simulink model "Kalman_compatible"  (R2021a)
settings: Solver=VariableStepAuto  StartTime=0.0  StopTime=10.0  RelTol=1e-3
values from neighbouring files (symbols this model uses):
  all_cov = cov(all_data)    [Analyze.m]
  ff = 1.1    [Analyze.m]
  g = 9.8    [Analyze.m]
  ground_alt = mean(z_hypsometric(ground_pressure))    [Analyze.m]
  T_s = 1/f_s    (= 0.005)    [Analyze.m]
undefined symbols (not defined in the file or in its folder): Aileron_A, Aileron_B, Discrete, Elevator_A, Elevator_B, Time
libraries: ctrlSharedLib x8
settings Model: Creator=jtc12  LastModifiedBy=Willi

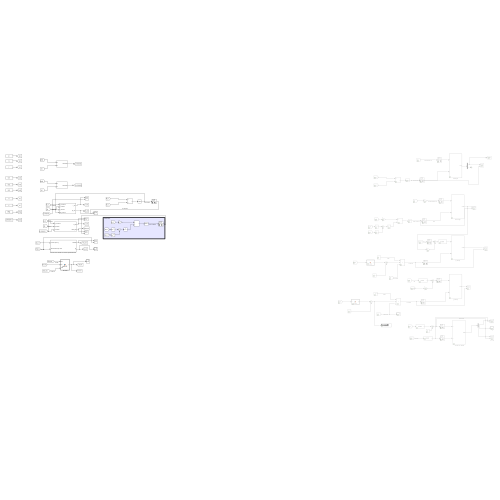
[thumbnail: Simulink's stored preview of the top-level diagram]
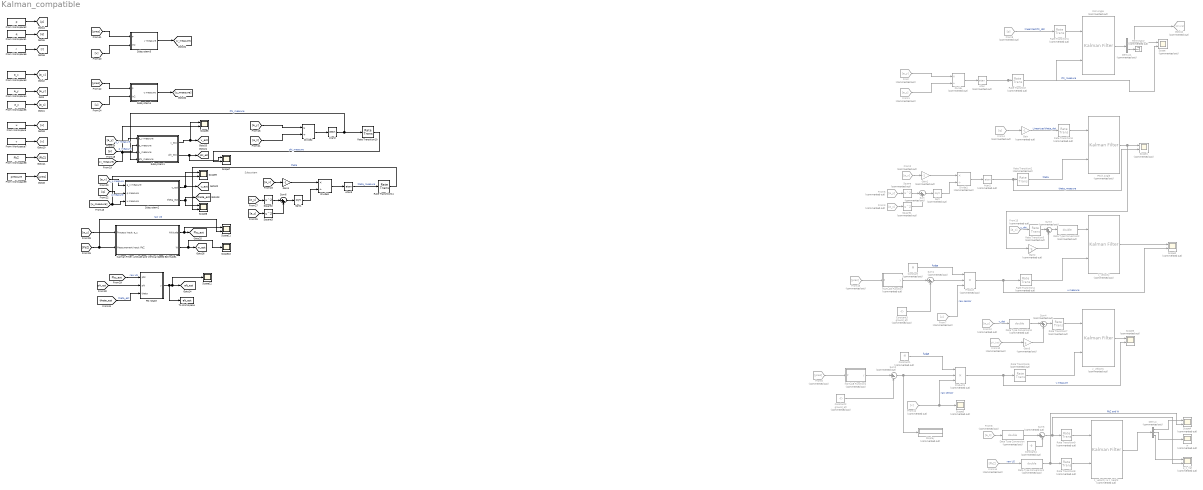
== system Kalman_compatible ==
  note: Subsystem
  Atan : Trigonometry  Commented=on  Operator=atan
  Atan1 : Trigonometry  Commented=on  Operator=atan
  Atan2 : Trigonometry  Operator=atan
  Atan3 : Trigonometry  Operator=atan
  Constant : Constant  Commented=on  Value=ff
  Constant1 : Constant  Commented=on  Value=ff
  Constant2 : Constant  Commented=on  Value=ground_alt
  Constant3 : Constant  Commented=on  Value=ground_alt
  Constant4 : Constant  Commented=on  Value=-9
  Data Type Conversion{,1..3} (4 alike) : DataTypeConversion  Commented=on  OutDataTypeStr=double
  Demux : Demux  Commented=on  Outputs=3
  Demux1 : Demux  Commented=on  Outputs=2
  Display : Display  Commented=on
  Divide : Product  Commented=on  Inputs=*/
  Divide1 : Product  Commented=on  Inputs=*/
  Divide2 : Product  Inputs=*/
  Divide3 : Product  Inputs=*/
  From : From  Commented=on  GotoTag=a_y
  From Workspace : FromWorkspace  VariableName=u
  From Workspace1 : FromWorkspace  VariableName=q
  From Workspace2 : FromWorkspace  VariableName=p
  From Workspace3 : FromWorkspace  VariableName=a_x
  From Workspace4 : FromWorkspace  VariableName=a_y
  From Workspace5 : FromWorkspace  VariableName=a_z
  From Workspace6 : FromWorkspace  VariableName=r
  From Workspace7 : FromWorkspace  VariableName=v
  From Workspace8 : FromWorkspace  VariableName=PbZ
  From Workspace9 : FromWorkspace  VariableName=pressure
  From1 : From  Commented=on  GotoTag=a_z
  From10 : From  Commented=on  GotoTag=phi_hat
  From11 : From  Commented=on  GotoTag=v
  From12 : From  Commented=on  GotoTag=a_y
  From13 : From  Commented=on  GotoTag=a_x
  From14 : From  Commented=on  GotoTag=PbZ
  From15 : From  Commented=on  GotoTag=pres
  From2 : From  Commented=on  GotoTag=a_x
  From3 : From  Commented=on  GotoTag=a_z
  From4 : From  Commented=on  GotoTag=q
  From5 : From  Commented=on  GotoTag=a_y
  From6 : From  Commented=on  GotoTag=pres
  From7 : From  Commented=on  GotoTag=u
  From8 : From  Commented=on  GotoTag=a_z
  From9 : From  Commented=on  GotoTag=p
  Gain : Gain  Commented=on  Gain=-1
  Gain1 : Gain  Commented=on  Gain=-1
  Gain2 : Gain  Commented=on  Gain=-g
  Gain3 : Gain  Commented=on  Gain=g
  Gain4 : Gain  Gain=-1
  Goto12 : Goto  Commented=on  GotoTag=phi_hat
  Kalman Filter: Altitude and Vertical Speed Estimate1 : Subsystem
  MATLAB Function : MATLAB Function  Commented=on  TreatAsAtomicUnit=on
  MATLAB Function1 : MATLAB Function  Commented=on  TreatAsAtomicUnit=on
  PD rotate : MATLAB Function  TreatAsAtomicUnit=on
  Pitch Angle : ctrlSharedLib/Kalman Filter  Commented=on  TimeDomain=Discrete-Time  UseCurrentEstimator=on  ModelSource=Individual A, B, C, D matrices  ModelSourceVariable=ss(0.95,1,1,0,1)  A=[1]  B=[1/200]  C=[1]  D=0  NumberOfStates=1  NumberOfInputs=1  NumberOfOutputs=1  InitialEstimateSource=Dialog  X0=0  P0=10  UseK=off  UseGH=off  NumberOfProcessNoiseInputs=1  G=1  TimeInvariantG=on  H=0  TimeInvariantH=on  Q=.0085/1000  TimeInvariantQ=on  R=.0066/10  TimeInvariantR=on  N=0  TimeInvariantN=on  AddInputPort=on  AddEnablePort=off  OutputEstimatedY=off  OutputP=off  Ts=-1
  Product : Product  Commented=on  Inputs=3
  Product1 : Product  Commented=on  Inputs=3
  Rate Transition{,1..9} (10 alike) : RateTransition  Commented=on  OutPortSampleTime=1/200
  Rate Transition10 : RateTransition  OutPortSampleTime=1/200
  Rate Transition11 : RateTransition  OutPortSampleTime=1/200
  Roll Angle : ctrlSharedLib/Kalman Filter  Commented=on  TimeDomain=Discrete-Time  UseCurrentEstimator=on  ModelSource=Individual A, B, C, D matrices  ModelSourceVariable=ss(0.95,1,1,0,1)  A=[1 1/200;0 1]  B=[0;1/200]  C=[1 0]  D=0  NumberOfStates=1  NumberOfInputs=1  NumberOfOutputs=1  InitialEstimateSource=Dialog  X0=0  P0=10  UseK=off  UseGH=off  NumberOfProcessNoiseInputs=1  G=1  TimeInvariantG=on  H=0  TimeInvariantH=on  Q=.0133/200  TimeInvariantQ=on  R=.0101  TimeInvariantR=on  N=0  TimeInvariantN=on  AddInputPort=on  AddEnablePort=off  OutputEstimatedY=off  OutputP=off  Ts=-1
  Scope{,1..4} (5 alike) : Scope  Commented=on  NumInputPorts=2
  Scope10 : Scope
  Scope{6..9,11} (5 alike) : Scope  NumInputPorts=2
  Scope12 : Scope
  Scope5 : Scope  Commented=on
  Sqrt : Sqrt  Commented=on  SaturateOnIntegerOverflow=on
  Sqrt1 : Sqrt  SaturateOnIntegerOverflow=on
  Square : Math  Commented=on  Operator=square  SaturateOnIntegerOverflow=on
  Square1 : Math  Commented=on  Operator=square  SaturateOnIntegerOverflow=on
  Square2 : Math  Operator=square  SaturateOnIntegerOverflow=on
  Square3 : Math  Operator=square  SaturateOnIntegerOverflow=on
  Subsystem1 : Subsystem
  Subsystem2 : Subsystem
  Subsystem3 : Subsystem
  Subsystem4 : Subsystem
  Sum : Sum  Commented=on  Inputs=|++
  Sum1 : Sum  Commented=on  Inputs=|+-
  Sum2 : Sum  Commented=on  Inputs=|+-
  Sum3 : Sum  Commented=on  Inputs=|++
  Sum4 : Sum  Commented=on  Inputs=|++
  Sum5 : Sum  Commented=on  Inputs=|+-
  Sum6 : Sum  Inputs=|++
  Terminator : Terminator  Commented=on
  To Workspace : ToWorkspace  VariableName=alt_est  SaveFormat=Structure With Time  SampleTime=-1
  a_z_hat : Scope  Commented=on  NumInputPorts=2
  w : Scope  Commented=on
  x_velocity : ctrlSharedLib/Kalman Filter  Commented=on  TimeDomain=Discrete-Time  UseCurrentEstimator=on  ModelSource=Individual A, B, C, D matrices  ModelSourceVariable=ss(0.95,1,1,0,1)  A=[1 1/200;0 1]  B=[0;1/200]  C=[1 0]  D=0  NumberOfStates=1  NumberOfInputs=1  NumberOfOutputs=1  InitialEstimateSource=Dialog  X0=0  P0=10  UseK=off  UseGH=off  NumberOfProcessNoiseInputs=1  G=1  TimeInvariantG=on  H=0  TimeInvariantH=on  Q=.0059/200  TimeInvariantQ=on  R=all_cov(10,8)*20  TimeInvariantR=on  N=0  TimeInvariantN=on  AddInputPort=on  AddEnablePort=off  OutputEstimatedY=off  OutputP=off  Ts=-1
  y_velocity : ctrlSharedLib/Kalman Filter  Commented=on  TimeDomain=Discrete-Time  UseCurrentEstimator=on  ModelSource=Individual A, B, C, D matrices  ModelSourceVariable=ss(0.95,1,1,0,1)  A=[1 1/200;0 1]  B=[0;1/200]  C=[1 0]  D=0  NumberOfStates=1  NumberOfInputs=1  NumberOfOutputs=1  InitialEstimateSource=Dialog  X0=0  P0=10  UseK=off  UseGH=off  NumberOfProcessNoiseInputs=1  G=1  TimeInvariantG=on  H=0  TimeInvariantH=on  Q=.0087/200  TimeInvariantQ=on  R=2.5  TimeInvariantR=on  N=0  TimeInvariantN=on  AddInputPort=on  AddEnablePort=off  OutputEstimatedY=off  OutputP=off  Ts=-1
  z_velocity & z_height : ctrlSharedLib/Kalman Filter  Commented=on  TimeDomain=Discrete-Time  UseCurrentEstimator=on  ModelSource=Individual A, B, C, D matrices  ModelSourceVariable=ss(0.95,1,1,0,1)  A=[1 1/200 0;0 1 1/200;0 0 1]  B=[0; 0; 1/200]  C=[1 0 0]  D=0  NumberOfStates=1  NumberOfInputs=1  NumberOfOutputs=1  InitialEstimateSource=Dialog  X0=0  P0=10  UseK=off  UseGH=off  NumberOfProcessNoiseInputs=1  G=1  TimeInvariantG=on  H=0  TimeInvariantH=on  Q=all_cov(7,7)/1000  TimeInvariantQ=on  R=all_cov(1,1)*50  TimeInvariantR=on  N=0  TimeInvariantN=on  AddInputPort=on  AddEnablePort=off  OutputEstimatedY=off  OutputP=off  Ts=-1
  tag scope: Pbz_est=global, alt_est=global, phi_est=global, theta_est=global, u_est=global, v_est=global, w_est=global
  wires:
  From/1 -> Divide/1
  From1/1 -> Divide/2
  Divide/1 -> Atan/1
  From Workspace3/1 -> [a_x]
  From Workspace4/1 -> [a_y]
  From Workspace5/1 -> [a_z]
  Atan/1 -> Scope/2, Rate Transition/1  "Phi_measure"
  Rate Transition/1 -> Roll Angle/2
  From Workspace2/1 -> [p]
  From Workspace1/1 -> [q]
  From Workspace6/1 -> [r]
  Rate Transition1/1 -> Roll Angle/1
  From9/1 -> Rate Transition1/1  "linearized Phi_dot"
  Atan1/1 -> Scope1/2, Rate Transition2/1  "theta_measure"
  Rate Transition2/1 -> Pitch Angle/2  "theta"
  Rate Transition3/1 -> Pitch Angle/1
  Pitch Angle/1 -> Gain2/1, Scope1/1
  Divide1/1 -> Atan1/1
  From4/1 -> Gain/1
  Gain/1 -> Rate Transition3/1  "Linearized theta_dot"
  From2/1 -> Gain1/1
  Gain1/1 -> Divide1/1
  From5/1 -> Square/1
  From3/1 -> Square1/1
  Square/1 -> Sum/1
  Square1/1 -> Sum/2
  Sum/1 -> Sqrt/1
  Sqrt/1 -> Divide1/2
  Rate Transition4/1 -> x_velocity/2
  From Workspace/1 -> [u]
  From Workspace7/1 -> [v]
  From Workspace8/1 -> [PbZ]
  Constant/1 -> Product/1  "fudge"
  From7/1 -> Product/3  "raw sensor"
  Product/1 -> Scope2/2, Rate Transition4/1  "u measure"
  Rate Transition7/1 -> y_velocity/1
  y_velocity/1 -> Scope3/1
  Product1/1 -> Rate Transition6/1, Scope3/2  "v measure"
  Rate Transition6/1 -> y_velocity/2
  Constant1/1 -> Product1/1  "fudge"
  From11/1 -> Product1/3, Scope5/1  "raw sensor"
  From13/1 -> Rate Transition5/1  "u_dot"
  Rate Transition8/1 -> z_velocity & z_height/2
  Rate Transition9/1 -> z_velocity & z_height/1
  From8/1 -> Data Type Conversion/1
  Data Type Conversion1/1 -> Scope4/2, Rate Transition8/1  "PbZ and W"
  From14/1 -> Data Type Conversion1/1  "raw US"
  Data Type Conversion2/1 -> x_velocity/1
  From12/1 -> Data Type Conversion3/1  "v_dot"
  From Workspace9/1 -> [pres]
  From15/1 -> MATLAB Function/1(P)
  Sum2/1 -> Display/1, Product1/2
  Sum1/1 -> Product/2
  MATLAB Function/1(y) -> Sum1/1
  Constant3/1 -> Sum1/2
  Constant2/1 -> Sum2/2
  MATLAB Function1/1(y) -> Sum2/1
  From6/1 -> MATLAB Function1/1(P)
  Sum3/1 -> Data Type Conversion2/1
  Rate Transition5/1 -> Sum3/1
  Gain2/1 -> Sum3/2
  Data Type Conversion3/1 -> Sum4/1
  Sum4/1 -> Rate Transition7/1
  Gain3/1 -> Sum4/2
  From10/1 -> Gain3/1
  Constant4/1 -> Sum5/2
  Demux/1 -> Scope4/1
  Demux/2 -> w/1
  z_velocity & z_height/1 -> Demux/1
  Roll Angle/1 -> Demux1/1
  Demux1/2 -> Terminator/1
  Demux1/1 -> Goto12/1, Scope/1
  x_velocity/1 -> Scope2/1
  Demux/3 -> a_z_hat/1
  Data Type Conversion/1 -> Sum5/1
  Sum5/1 -> a_z_hat/2, Rate Transition9/1
  Subsystem2/2(theta_est) -> Scope8/1, [theta_est]
  [a_x] -> Subsystem2/1(a_x measure)  "a_x measure"
  [q] -> Subsystem2/2(q measure)  "q measure"
  Subsystem2/1(u_est) -> Scope9/1, [u_est]
  [v] -> Subsystem3/2(In2)
  Subsystem4/1(u measure) -> [u_measure]
  [pres] -> Subsystem4/1(P)
  [v_measure] -> Scope6/2, Subsystem1/3(v_measure)
  [u_measure] -> Scope9/2, Subsystem2/3(u measure)
  Subsystem1/1(v_est) -> Scope6/1, [v_est]
  [p] -> Subsystem1/2(p_measure)  "p_measure"
  [a_y] -> Subsystem1/1(a_y measure)  "a_y measure"
  [u] -> Subsystem4/2(In2)
  [pres] -> Subsystem3/1(P)
  [phi_est] -> PD rotate/2(phi)
  PD rotate/1(y) -> To Workspace/1, Scope12/1, [alt_est]
  [theta_est] -> PD rotate/3(theta)  "theta_est"
  [PbZ] -> Scope11/2, Kalman Filter: Altitude and Vertical Speed Estimate1/2(Measurement Input: PbZ)  "raw US"
  [Pbz_est] -> PD rotate/1(pbz)  "raw US"
  Kalman Filter: Altitude and Vertical Speed Estimate1/1(Altitude) -> Scope11/1, [Pbz_est]
  Kalman Filter: Altitude and Vertical Speed Estimate1/2(W) -> Scope10/1, [w_est]
  Subsystem3/1(v measure) -> [v_measure]
  [a_z] -> Kalman Filter: Altitude and Vertical Speed Estimate1/1("Process Input: a_z ")
  Subsystem1/2(phi_est) -> Scope7/1, [phi_est]
  Divide2/1 -> Atan2/1
  [a_z] -> Divide2/2
  Atan2/1 -> Subsystem1/4(phi_measure), Rate Transition10/1  "Phi_measure"
  [a_y] -> Divide2/1
  Rate Transition10/1 -> Scope7/2  "phi_measure"
  Rate Transition11/1 -> Scope8/2  "theta"
  Atan3/1 -> Rate Transition11/1  "theta_measure"
  [a_z] -> Square3/1
  Square2/1 -> Sum6/1
  [a_x] -> Gain4/1
  Sum6/1 -> Sqrt1/1
  Sqrt1/1 -> Divide3/2
  Gain4/1 -> Divide3/1
  Divide3/1 -> Atan3/1
  Square3/1 -> Sum6/2
  [a_y] -> Square2/1

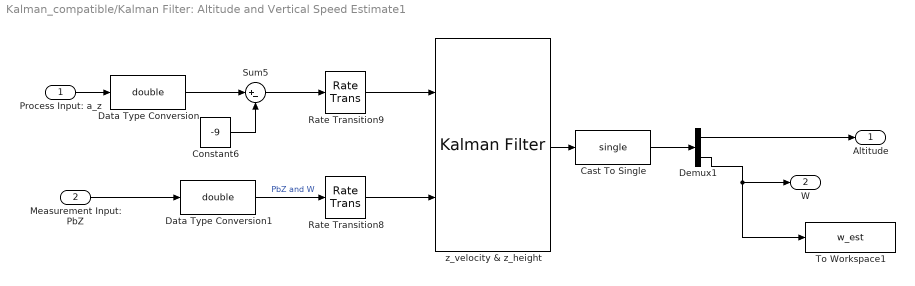
== system Kalman_compatible/Kalman Filter: Altitude and Vertical Speed Estimate1 ==
  "Process Input: a_z " : Inport
  Measurement Input: PbZ : Inport  Port=2
  Cast To Single : DataTypeConversion  OutDataTypeStr=single
  Constant6 : Constant  Value=-9
  Data Type Conversion : DataTypeConversion  OutDataTypeStr=double
  Data Type Conversion1 : DataTypeConversion  OutDataTypeStr=double
  Demux1 : Demux  Outputs=2
  Rate Transition8 : RateTransition  OutPortSampleTime=1/200
  Rate Transition9 : RateTransition  OutPortSampleTime=1/200
  Sum5 : Sum  Inputs=|+-
  To Workspace1 : ToWorkspace  VariableName=w_est  SaveFormat=Structure With Time  SampleTime=-1
  z_velocity & z_height : ctrlSharedLib/Kalman Filter  TimeDomain=Discrete-Time  UseCurrentEstimator=on  ModelSource=Individual A, B, C, D matrices  ModelSourceVariable=ss(0.95,1,1,0,1)  A=[1 1/200;0 1]  B=[0; 1/200]  C=[1 0]  D=0  NumberOfStates=1  NumberOfInputs=1  NumberOfOutputs=1  InitialEstimateSource=Dialog  X0=0  P0=10  UseK=off  UseGH=off  NumberOfProcessNoiseInputs=1  G=1  TimeInvariantG=on  H=0  TimeInvariantH=on  Q=all_cov(7,7)/1000  TimeInvariantQ=on  R=all_cov(1,1)*50  TimeInvariantR=on  N=0  TimeInvariantN=on  AddInputPort=on  AddEnablePort=off  OutputEstimatedY=off  OutputP=off  Ts=-1
  Altitude : Outport
  W : Outport  Port=2
  wires:
  Data Type Conversion1/1 -> Rate Transition8/1  "PbZ and W"
  Constant6/1 -> Sum5/2
  Demux1/1 -> Altitude/1
  z_velocity & z_height/1 -> Cast To Single/1
  Sum5/1 -> Rate Transition9/1
  Data Type Conversion/1 -> Sum5/1
  Rate Transition9/1 -> z_velocity & z_height/1
  Rate Transition8/1 -> z_velocity & z_height/2
  Measurement Input: PbZ/1 -> Data Type Conversion1/1
  Demux1/2 -> W/1, To Workspace1/1
  "Process Input: a_z "/1 -> Data Type Conversion/1
  Cast To Single/1 -> Demux1/1

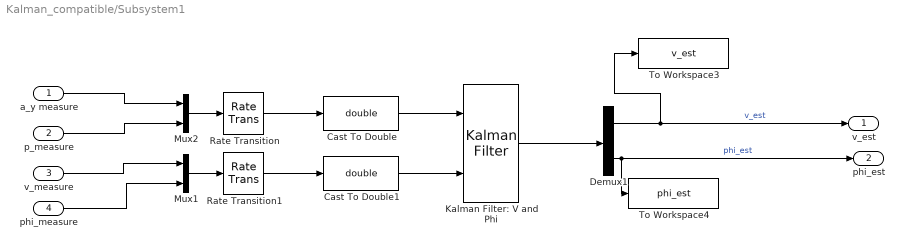
== system Kalman_compatible/Subsystem1 ==
  a_y measure : Inport
  p_measure : Inport  Port=2
  v_measure : Inport  Port=3
  phi_measure : Inport  Port=4
  Cast To Double : DataTypeConversion  OutDataTypeStr=double
  Cast To Double1 : DataTypeConversion  OutDataTypeStr=double
  Demux1 : Demux  Outputs=2
  Kalman Filter: V and Phi : ctrlSharedLib/Kalman Filter  TimeDomain=Discrete-Time  UseCurrentEstimator=on  ModelSource=Individual A, B, C, D matrices  ModelSourceVariable=ss(0.95,1,1,0,1)  A=Aileron_A  B=Aileron_B  C=eye(2)  D=0  NumberOfStates=1  NumberOfInputs=1  NumberOfOutputs=1  InitialEstimateSource=Dialog  X0=0  P0=10  UseK=off  UseGH=off  NumberOfProcessNoiseInputs=1  G=1  TimeInvariantG=on  H=0  TimeInvariantH=on  Q=[all_cov(6,6) all_cov(6,2); all_cov(2,6) all_cov(2,2)]*T_s  TimeInvariantQ=on  R=[all_cov(9,9) all_cov(9,6)*all_cov(9,7);all_cov(9,6)*all_cov(9,7) all_cov(6,6)*all_cov(7,7)]*1000  TimeInvariantR=on  N=0  TimeInvariantN=on  AddInputPort=on  AddEnablePort=off  OutputEstimatedY=off  OutputP=off  Ts=-1
  Mux1 : Mux  Inputs=2
  Mux2 : Mux  Inputs=2
  Rate Transition : RateTransition  OutPortSampleTime=1/200
  Rate Transition1 : RateTransition  OutPortSampleTime=1/200
  To Workspace3 : ToWorkspace  VariableName=v_est  SaveFormat=Structure With Time  SampleTime=-1
  To Workspace4 : ToWorkspace  VariableName=phi_est  SaveFormat=Structure With Time  SampleTime=-1
  v_est : Outport
  phi_est : Outport  Port=2
  wires:
  Rate Transition/1 -> Cast To Double/1
  Mux2/1 -> Rate Transition/1
  Rate Transition1/1 -> Cast To Double1/1
  Demux1/2 -> phi_est/1, To Workspace4/1  "phi_est"
  Kalman Filter: V and Phi/1 -> Demux1/1
  Demux1/1 -> v_est/1, To Workspace3/1  "v_est"
  a_y measure/1 -> Mux2/1
  p_measure/1 -> Mux2/2
  Cast To Double/1 -> Kalman Filter: V and Phi/1
  Cast To Double1/1 -> Kalman Filter: V and Phi/2
  Mux1/1 -> Rate Transition1/1
  v_measure/1 -> Mux1/1
  phi_measure/1 -> Mux1/2

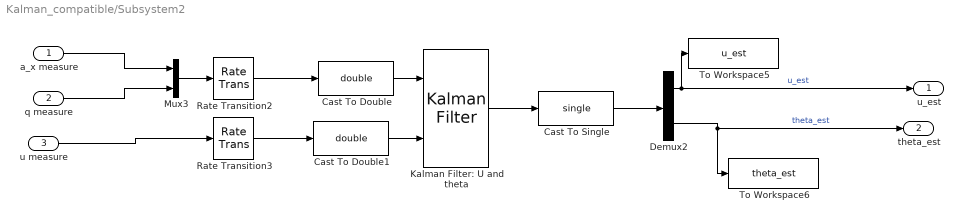
== system Kalman_compatible/Subsystem2 ==
  a_x measure : Inport
  q measure : Inport  Port=2
  u measure : Inport  Port=3
  Cast To Double : DataTypeConversion  OutDataTypeStr=double
  Cast To Double1 : DataTypeConversion  OutDataTypeStr=double
  Cast To Single : DataTypeConversion  OutDataTypeStr=single
  Demux2 : Demux  Outputs=2
  Kalman Filter: U and theta : ctrlSharedLib/Kalman Filter  TimeDomain=Discrete-Time  UseCurrentEstimator=on  ModelSource=Individual A, B, C, D matrices  ModelSourceVariable=ss(0.95,1,1,0,1)  A=Elevator_A  B=Elevator_B  C=[1 0]  D=0  NumberOfStates=1  NumberOfInputs=1  NumberOfOutputs=1  InitialEstimateSource=Dialog  X0=0  P0=10  UseK=off  UseGH=off  NumberOfProcessNoiseInputs=1  G=1  TimeInvariantG=on  H=0  TimeInvariantH=on  Q=[all_cov(5,5) all_cov(5,2); all_cov(2,5) all_cov(2,2)]*T_s  TimeInvariantQ=on  R=all_cov(8,8)*10000  TimeInvariantR=on  N=0  TimeInvariantN=on  AddInputPort=on  AddEnablePort=off  OutputEstimatedY=off  OutputP=off  Ts=-1
  Mux3 : Mux  Inputs=2
  Rate Transition2 : RateTransition  OutPortSampleTime=1/200
  Rate Transition3 : RateTransition  OutPortSampleTime=1/200
  To Workspace5 : ToWorkspace  VariableName=u_est  SaveFormat=Structure With Time  SampleTime=-1
  To Workspace6 : ToWorkspace  VariableName=theta_est  SaveFormat=Structure With Time  SampleTime=-1
  u_est : Outport
  theta_est : Outport  Port=2
  wires:
  Mux3/1 -> Rate Transition2/1
  Rate Transition3/1 -> Cast To Double1/1
  Rate Transition2/1 -> Cast To Double/1
  Demux2/2 -> theta_est/1, To Workspace6/1  "theta_est"
  Demux2/1 -> u_est/1, To Workspace5/1  "u_est"
  q measure/1 -> Mux3/2
  u measure/1 -> Rate Transition3/1
  Kalman Filter: U and theta/1 -> Cast To Single/1
  a_x measure/1 -> Mux3/1
  Cast To Double/1 -> Kalman Filter: U and theta/1
  Cast To Double1/1 -> Kalman Filter: U and theta/2
  Cast To Single/1 -> Demux2/1

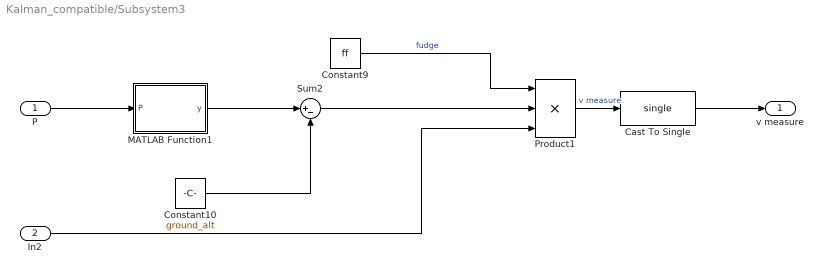
== system Kalman_compatible/Subsystem3 ==
  P : Inport
  In2 : Inport  Port=2
  Cast To Single : DataTypeConversion  OutDataTypeStr=single
  Constant10 : Constant  Value=ground_alt
  Constant9 : Constant  Value=ff
  MATLAB Function1 : MATLAB Function  TreatAsAtomicUnit=on
  Product1 : Product  Inputs=3
  Sum2 : Sum  Inputs=|+-
  v measure : Outport
  wires:
  Sum2/1 -> Product1/2
  Constant10/1 -> Sum2/2
  P/1 -> MATLAB Function1/1(P)
  Product1/1 -> Cast To Single/1  "v measure"
  Constant9/1 -> Product1/1  "fudge"
  MATLAB Function1/1(y) -> Sum2/1
  In2/1 -> Product1/3
  Cast To Single/1 -> v measure/1

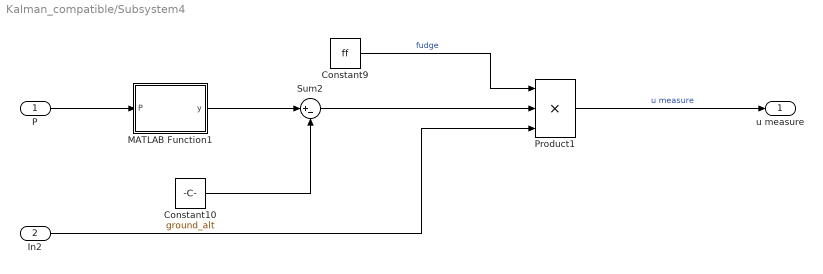
== system Kalman_compatible/Subsystem4 ==
  P : Inport
  In2 : Inport  Port=2
  Constant10 : Constant  Value=ground_alt
  Constant9 : Constant  Value=ff
  MATLAB Function1 : MATLAB Function  TreatAsAtomicUnit=on
  Product1 : Product  Inputs=3
  Sum2 : Sum  Inputs=|+-
  u measure : Outport
  wires:
  Sum2/1 -> Product1/2
  Constant10/1 -> Sum2/2
  P/1 -> MATLAB Function1/1(P)
  Product1/1 -> u measure/1  "u measure"
  Constant9/1 -> Product1/1  "fudge"
  MATLAB Function1/1(y) -> Sum2/1
  In2/1 -> Product1/3

== matlab function Kalman_compatible/MATLAB Function ==
  data: P input; y output
function y = z_pres(P)
g = 9.8; % acceleration due to gravity m/s^2
M = 0.0289644; % molar mass of air in kg/mol
R = 8.31432; % universal gas constant Nm/mol/k
p0 = 101325; % Pa standard pressure

T =288.15;  % Assumed temperature in kelvin
K =-g*M/R/T;
z_hypsometric = 1/K*log(P/p0);
y = z_hypsometric;

== matlab function Kalman_compatible/PD rotate ==
  data: pbz input; y output; phi input; theta input
function y = rotate_BE(pbz, phi, theta)
roll_BE = [1 0 0; 0 cos(phi) sin(phi); 0 -sin(phi) cos(phi)]';
pitch_BE = [cos(theta) 0 -sin(theta); 0 1 0; sin(theta) 0 cos(theta);]';
%yaw_BE = simplify(inv([cos(psi) sin(psi) 0; -sin(psi) cos(psi) 0; 0 0 1;]));
rotater = roll_BE*pitch_BE*pbz;
y = rotater(3);

== matlab function Kalman_compatible/Subsystem3/MATLAB Function1 ==
  data: P input; y output
function y = z_pres(P)
g = 9.8; % acceleration due to gravity m/s^2
M = 0.0289644; % molar mass of air in kg/mol
R = 8.31432; % universal gas constant Nm/mol/k
p0 = 101325; % Pa standard pressure

T =288.15;  % Assumed temperature in kelvin
K =-g*M/R/T;
z_hypsometric = 1/K*log(P/p0);
y = z_hypsometric;

== matlab function Kalman_compatible/Subsystem4/MATLAB Function1 ==
  data: P input; y output
function y = z_pres(P)
g = 9.8; % acceleration due to gravity m/s^2
M = 0.0289644; % molar mass of air in kg/mol
R = 8.31432; % universal gas constant Nm/mol/k
p0 = 101325; % Pa standard pressure

T =288.15;  % Assumed temperature in kelvin
K =-g*M/R/T;
z_hypsometric = 1/K*log(P/p0);
y = z_hypsometric;

== matlab function Kalman_compatible/MATLAB Function1 ==
  data: P input; y output
function y = z_pres(P)
g = 9.8; % acceleration due to gravity m/s^2
M = 0.0289644; % molar mass of air in kg/mol
R = 8.31432; % universal gas constant Nm/mol/k
p0 = 101325; % Pa standard pressure

T =288.15;  % Assumed temperature in kelvin
K =-g*M/R/T;
z_hypsometric = 1/K*log(P/p0);
y = z_hypsometric;
